simulink model "AdaptiveDilterPrototype"  (R2022b)
settings: Solver=VariableStepAuto  StartTime=0.0  StopTime=10.0  RelTol=1e-3
settings Model: Creator=Ceribro  LastModifiedBy=Ceribro

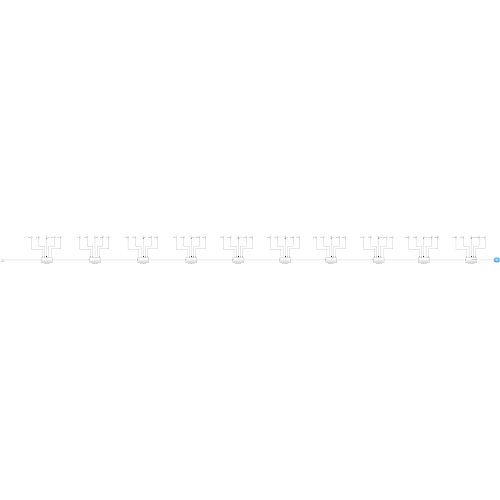
[thumbnail: Simulink's stored preview of the top-level diagram]
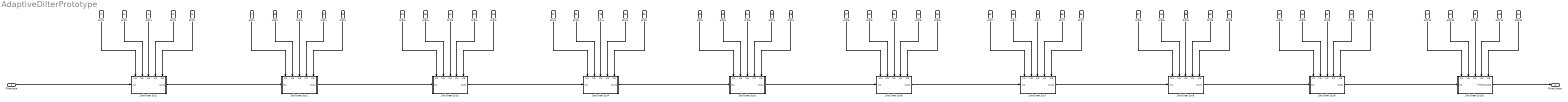
== system AdaptiveDilterPrototype ==
  FilterInput : Inport
  a(2)1 : Inport  Port=2
  b(2)1 : Inport  Port=3
  b(1)1 : Inport  Port=4
  a(3)1 : Inport  Port=5
  b(3)1 : Inport  Port=6
  a(2)2 : Inport  Port=7
  b(2)2 : Inport  Port=8
  b(1)2 : Inport  Port=9
  a(3)2 : Inport  Port=10
  b(3)2 : Inport  Port=11
  a(2)3 : Inport  Port=12
  b(2)3 : Inport  Port=13
  b(1)3 : Inport  Port=14
  a(3)3 : Inport  Port=15
  b(3)3 : Inport  Port=16
  a(2)4 : Inport  Port=17
  b(2)4 : Inport  Port=18
  b(1)4 : Inport  Port=19
  a(3)4 : Inport  Port=20
  b(3)4 : Inport  Port=21
  a(2)5 : Inport  Port=22
  b(2)5 : Inport  Port=23
  b(1)5 : Inport  Port=24
  a(3)5 : Inport  Port=25
  b(3)5 : Inport  Port=26
  a(2)6 : Inport  Port=27
  b(2)6 : Inport  Port=28
  b(1)6 : Inport  Port=29
  a(3)6 : Inport  Port=30
  b(3)6 : Inport  Port=31
  a(2)7 : Inport  Port=32
  b(2)7 : Inport  Port=33
  b(1)7 : Inport  Port=34
  a(3)7 : Inport  Port=35
  b(3)7 : Inport  Port=36
  a(2)8 : Inport  Port=37
  b(2)8 : Inport  Port=38
  b(1)8 : Inport  Port=39
  a(3)8 : Inport  Port=40
  b(3)8 : Inport  Port=41
  a(2)9 : Inport  Port=42
  b(2)9 : Inport  Port=43
  b(1)9 : Inport  Port=44
  a(3)9 : Inport  Port=45
  b(3)9 : Inport  Port=46
  a(2)10 : Inport  Port=47
  b(2)10 : Inport  Port=48
  b(1)10 : Inport  Port=49
  a(3)10 : Inport  Port=50
  b(3)10 : Inport  Port=51
  2nd Order Sys1 : Subsystem
      settings: PortSchema="{\"entries\":[{\"content\":{\"sides\":[{\"content\":{\"connectorIds\":[\"In1\",\"In2\",\"In3\",\"In4\",\"In5\"]},\"type\":\"ConnectorPlacement.EquallySpacedRectSide\",\"uuid\":\"b9dbb1a8-51a6-4b96-96bf-c9da2300ff43\"},{\"content\":{\"connectorIds\":[],\"side\":\"RIGHT\"},\"type\":\"ConnectorPlacement.EquallySpacedRectSide\",\"uuid\":\"4cac1354-1c5d-4db6-b4d6-5d3a283dca26\"},{\"content\":{\"connectorIds\":[\"In6\"],\"side\":\"TOP\"},\"type\":\"ConnectorPlacement.EquallySpacedRectSide\",\"uuid\":\"b7090e22-aad0-44be-a576-af352fa4e03b\"},{\"content\":{\"connectorIds\":[\"Out1\"],\"side\":\"BOTTOM\"},\"type\":\"ConnectorPlacement.EquallySpacedRectSide\",\"uuid\":\"8692f441-cf04-4506-bf52-8e3a9e9e20b6\"}]},\"type\":\"ConnectorPlacement.EquallySpacedConnector\",\"uuid\":\"e0d2a6b7-a198-4ea6-960b-9fb200603ab4\"}],\"packageUris\":[\"http://schema.mathworks.com/mf0/Connector/R2020b\"],\"version\":\"1.0\"}"
  2nd Order Sys10 : Subsystem
      settings: PortSchema="{\"entries\":[{\"content\":{\"sides\":[{\"content\":{\"connectorIds\":[\"In1\",\"In2\",\"In3\",\"In4\",\"In5\"]},\"type\":\"ConnectorPlacement.EquallySpacedRectSide\",\"uuid\":\"b9dbb1a8-51a6-4b96-96bf-c9da2300ff43\"},{\"content\":{\"connectorIds\":[],\"side\":\"RIGHT\"},\"type\":\"ConnectorPlacement.EquallySpacedRectSide\",\"uuid\":\"4cac1354-1c5d-4db6-b4d6-5d3a283dca26\"},{\"content\":{\"connectorIds\":[\"In6\"],\"side\":\"TOP\"},\"type\":\"ConnectorPlacement.EquallySpacedRectSide\",\"uuid\":\"b7090e22-aad0-44be-a576-af352fa4e03b\"},{\"content\":{\"connectorIds\":[\"Out1\"],\"side\":\"BOTTOM\"},\"type\":\"ConnectorPlacement.EquallySpacedRectSide\",\"uuid\":\"8692f441-cf04-4506-bf52-8e3a9e9e20b6\"}]},\"type\":\"ConnectorPlacement.EquallySpacedConnector\",\"uuid\":\"e0d2a6b7-a198-4ea6-960b-9fb200603ab4\"}],\"packageUris\":[\"http://schema.mathworks.com/mf0/Connector/R2020b\"],\"version\":\"1.0\"}"
  2nd Order Sys2 : Subsystem
      settings: PortSchema="{\"entries\":[{\"content\":{\"sides\":[{\"content\":{\"connectorIds\":[\"In1\",\"In2\",\"In3\",\"In4\",\"In5\"]},\"type\":\"ConnectorPlacement.EquallySpacedRectSide\",\"uuid\":\"b9dbb1a8-51a6-4b96-96bf-c9da2300ff43\"},{\"content\":{\"connectorIds\":[],\"side\":\"RIGHT\"},\"type\":\"ConnectorPlacement.EquallySpacedRectSide\",\"uuid\":\"4cac1354-1c5d-4db6-b4d6-5d3a283dca26\"},{\"content\":{\"connectorIds\":[\"In6\"],\"side\":\"TOP\"},\"type\":\"ConnectorPlacement.EquallySpacedRectSide\",\"uuid\":\"b7090e22-aad0-44be-a576-af352fa4e03b\"},{\"content\":{\"connectorIds\":[\"Out1\"],\"side\":\"BOTTOM\"},\"type\":\"ConnectorPlacement.EquallySpacedRectSide\",\"uuid\":\"8692f441-cf04-4506-bf52-8e3a9e9e20b6\"}]},\"type\":\"ConnectorPlacement.EquallySpacedConnector\",\"uuid\":\"e0d2a6b7-a198-4ea6-960b-9fb200603ab4\"}],\"packageUris\":[\"http://schema.mathworks.com/mf0/Connector/R2020b\"],\"version\":\"1.0\"}"
  2nd Order Sys3 : Subsystem
      settings: PortSchema="{\"entries\":[{\"content\":{\"sides\":[{\"content\":{\"connectorIds\":[\"In1\",\"In2\",\"In3\",\"In4\",\"In5\"]},\"type\":\"ConnectorPlacement.EquallySpacedRectSide\",\"uuid\":\"b9dbb1a8-51a6-4b96-96bf-c9da2300ff43\"},{\"content\":{\"connectorIds\":[],\"side\":\"RIGHT\"},\"type\":\"ConnectorPlacement.EquallySpacedRectSide\",\"uuid\":\"4cac1354-1c5d-4db6-b4d6-5d3a283dca26\"},{\"content\":{\"connectorIds\":[\"In6\"],\"side\":\"TOP\"},\"type\":\"ConnectorPlacement.EquallySpacedRectSide\",\"uuid\":\"b7090e22-aad0-44be-a576-af352fa4e03b\"},{\"content\":{\"connectorIds\":[\"Out1\"],\"side\":\"BOTTOM\"},\"type\":\"ConnectorPlacement.EquallySpacedRectSide\",\"uuid\":\"8692f441-cf04-4506-bf52-8e3a9e9e20b6\"}]},\"type\":\"ConnectorPlacement.EquallySpacedConnector\",\"uuid\":\"e0d2a6b7-a198-4ea6-960b-9fb200603ab4\"}],\"packageUris\":[\"http://schema.mathworks.com/mf0/Connector/R2020b\"],\"version\":\"1.0\"}"
  2nd Order Sys4 : Subsystem
      settings: PortSchema="{\"entries\":[{\"content\":{\"sides\":[{\"content\":{\"connectorIds\":[\"In1\",\"In2\",\"In3\",\"In4\",\"In5\"]},\"type\":\"ConnectorPlacement.EquallySpacedRectSide\",\"uuid\":\"b9dbb1a8-51a6-4b96-96bf-c9da2300ff43\"},{\"content\":{\"connectorIds\":[],\"side\":\"RIGHT\"},\"type\":\"ConnectorPlacement.EquallySpacedRectSide\",\"uuid\":\"4cac1354-1c5d-4db6-b4d6-5d3a283dca26\"},{\"content\":{\"connectorIds\":[\"In6\"],\"side\":\"TOP\"},\"type\":\"ConnectorPlacement.EquallySpacedRectSide\",\"uuid\":\"b7090e22-aad0-44be-a576-af352fa4e03b\"},{\"content\":{\"connectorIds\":[\"Out1\"],\"side\":\"BOTTOM\"},\"type\":\"ConnectorPlacement.EquallySpacedRectSide\",\"uuid\":\"8692f441-cf04-4506-bf52-8e3a9e9e20b6\"}]},\"type\":\"ConnectorPlacement.EquallySpacedConnector\",\"uuid\":\"e0d2a6b7-a198-4ea6-960b-9fb200603ab4\"}],\"packageUris\":[\"http://schema.mathworks.com/mf0/Connector/R2020b\"],\"version\":\"1.0\"}"
  2nd Order Sys5 : Subsystem
      settings: PortSchema="{\"entries\":[{\"content\":{\"sides\":[{\"content\":{\"connectorIds\":[\"In1\",\"In2\",\"In3\",\"In4\",\"In5\"]},\"type\":\"ConnectorPlacement.EquallySpacedRectSide\",\"uuid\":\"b9dbb1a8-51a6-4b96-96bf-c9da2300ff43\"},{\"content\":{\"connectorIds\":[],\"side\":\"RIGHT\"},\"type\":\"ConnectorPlacement.EquallySpacedRectSide\",\"uuid\":\"4cac1354-1c5d-4db6-b4d6-5d3a283dca26\"},{\"content\":{\"connectorIds\":[\"In6\"],\"side\":\"TOP\"},\"type\":\"ConnectorPlacement.EquallySpacedRectSide\",\"uuid\":\"b7090e22-aad0-44be-a576-af352fa4e03b\"},{\"content\":{\"connectorIds\":[\"Out1\"],\"side\":\"BOTTOM\"},\"type\":\"ConnectorPlacement.EquallySpacedRectSide\",\"uuid\":\"8692f441-cf04-4506-bf52-8e3a9e9e20b6\"}]},\"type\":\"ConnectorPlacement.EquallySpacedConnector\",\"uuid\":\"e0d2a6b7-a198-4ea6-960b-9fb200603ab4\"}],\"packageUris\":[\"http://schema.mathworks.com/mf0/Connector/R2020b\"],\"version\":\"1.0\"}"
  2nd Order Sys6 : Subsystem
      settings: PortSchema="{\"entries\":[{\"content\":{\"sides\":[{\"content\":{\"connectorIds\":[\"In1\",\"In2\",\"In3\",\"In4\",\"In5\"]},\"type\":\"ConnectorPlacement.EquallySpacedRectSide\",\"uuid\":\"b9dbb1a8-51a6-4b96-96bf-c9da2300ff43\"},{\"content\":{\"connectorIds\":[],\"side\":\"RIGHT\"},\"type\":\"ConnectorPlacement.EquallySpacedRectSide\",\"uuid\":\"4cac1354-1c5d-4db6-b4d6-5d3a283dca26\"},{\"content\":{\"connectorIds\":[\"In6\"],\"side\":\"TOP\"},\"type\":\"ConnectorPlacement.EquallySpacedRectSide\",\"uuid\":\"b7090e22-aad0-44be-a576-af352fa4e03b\"},{\"content\":{\"connectorIds\":[\"Out1\"],\"side\":\"BOTTOM\"},\"type\":\"ConnectorPlacement.EquallySpacedRectSide\",\"uuid\":\"8692f441-cf04-4506-bf52-8e3a9e9e20b6\"}]},\"type\":\"ConnectorPlacement.EquallySpacedConnector\",\"uuid\":\"e0d2a6b7-a198-4ea6-960b-9fb200603ab4\"}],\"packageUris\":[\"http://schema.mathworks.com/mf0/Connector/R2020b\"],\"version\":\"1.0\"}"
  2nd Order Sys7 : Subsystem
      settings: PortSchema="{\"entries\":[{\"content\":{\"sides\":[{\"content\":{\"connectorIds\":[\"In1\",\"In2\",\"In3\",\"In4\",\"In5\"]},\"type\":\"ConnectorPlacement.EquallySpacedRectSide\",\"uuid\":\"b9dbb1a8-51a6-4b96-96bf-c9da2300ff43\"},{\"content\":{\"connectorIds\":[],\"side\":\"RIGHT\"},\"type\":\"ConnectorPlacement.EquallySpacedRectSide\",\"uuid\":\"4cac1354-1c5d-4db6-b4d6-5d3a283dca26\"},{\"content\":{\"connectorIds\":[\"In6\"],\"side\":\"TOP\"},\"type\":\"ConnectorPlacement.EquallySpacedRectSide\",\"uuid\":\"b7090e22-aad0-44be-a576-af352fa4e03b\"},{\"content\":{\"connectorIds\":[\"Out1\"],\"side\":\"BOTTOM\"},\"type\":\"ConnectorPlacement.EquallySpacedRectSide\",\"uuid\":\"8692f441-cf04-4506-bf52-8e3a9e9e20b6\"}]},\"type\":\"ConnectorPlacement.EquallySpacedConnector\",\"uuid\":\"e0d2a6b7-a198-4ea6-960b-9fb200603ab4\"}],\"packageUris\":[\"http://schema.mathworks.com/mf0/Connector/R2020b\"],\"version\":\"1.0\"}"
  2nd Order Sys8 : Subsystem
      settings: PortSchema="{\"entries\":[{\"content\":{\"sides\":[{\"content\":{\"connectorIds\":[\"In1\",\"In2\",\"In3\",\"In4\",\"In5\"]},\"type\":\"ConnectorPlacement.EquallySpacedRectSide\",\"uuid\":\"b9dbb1a8-51a6-4b96-96bf-c9da2300ff43\"},{\"content\":{\"connectorIds\":[],\"side\":\"RIGHT\"},\"type\":\"ConnectorPlacement.EquallySpacedRectSide\",\"uuid\":\"4cac1354-1c5d-4db6-b4d6-5d3a283dca26\"},{\"content\":{\"connectorIds\":[\"In6\"],\"side\":\"TOP\"},\"type\":\"ConnectorPlacement.EquallySpacedRectSide\",\"uuid\":\"b7090e22-aad0-44be-a576-af352fa4e03b\"},{\"content\":{\"connectorIds\":[\"Out1\"],\"side\":\"BOTTOM\"},\"type\":\"ConnectorPlacement.EquallySpacedRectSide\",\"uuid\":\"8692f441-cf04-4506-bf52-8e3a9e9e20b6\"}]},\"type\":\"ConnectorPlacement.EquallySpacedConnector\",\"uuid\":\"e0d2a6b7-a198-4ea6-960b-9fb200603ab4\"}],\"packageUris\":[\"http://schema.mathworks.com/mf0/Connector/R2020b\"],\"version\":\"1.0\"}"
  2nd Order Sys9 : Subsystem
      settings: PortSchema="{\"entries\":[{\"content\":{\"sides\":[{\"content\":{\"connectorIds\":[\"In1\",\"In2\",\"In3\",\"In4\",\"In5\"]},\"type\":\"ConnectorPlacement.EquallySpacedRectSide\",\"uuid\":\"b9dbb1a8-51a6-4b96-96bf-c9da2300ff43\"},{\"content\":{\"connectorIds\":[],\"side\":\"RIGHT\"},\"type\":\"ConnectorPlacement.EquallySpacedRectSide\",\"uuid\":\"4cac1354-1c5d-4db6-b4d6-5d3a283dca26\"},{\"content\":{\"connectorIds\":[\"In6\"],\"side\":\"TOP\"},\"type\":\"ConnectorPlacement.EquallySpacedRectSide\",\"uuid\":\"b7090e22-aad0-44be-a576-af352fa4e03b\"},{\"content\":{\"connectorIds\":[\"Out1\"],\"side\":\"BOTTOM\"},\"type\":\"ConnectorPlacement.EquallySpacedRectSide\",\"uuid\":\"8692f441-cf04-4506-bf52-8e3a9e9e20b6\"}]},\"type\":\"ConnectorPlacement.EquallySpacedConnector\",\"uuid\":\"e0d2a6b7-a198-4ea6-960b-9fb200603ab4\"}],\"packageUris\":[\"http://schema.mathworks.com/mf0/Connector/R2020b\"],\"version\":\"1.0\"}"
  FilterOutput : Outport
  wires:
  a(2)1/1 -> 2nd Order Sys1/1(In1)
  b(2)1/1 -> 2nd Order Sys1/4(In2)
  b(1)1/1 -> 2nd Order Sys1/3(In3)
  FilterInput/1 -> 2nd Order Sys1/6(In4)
  a(3)1/1 -> 2nd Order Sys1/2(In5)
  b(3)1/1 -> 2nd Order Sys1/5(In6)
  a(3)2/1 -> 2nd Order Sys2/2(In5)
  2nd Order Sys1/1(Out1) -> 2nd Order Sys2/6(In4)
  b(2)2/1 -> 2nd Order Sys2/4(In2)
  b(1)2/1 -> 2nd Order Sys2/3(In3)
  a(2)2/1 -> 2nd Order Sys2/1(In1)
  b(3)2/1 -> 2nd Order Sys2/5(In6)
  a(2)3/1 -> 2nd Order Sys3/1(In1)
  b(2)3/1 -> 2nd Order Sys3/4(In2)
  b(3)3/1 -> 2nd Order Sys3/5(In6)
  a(3)3/1 -> 2nd Order Sys3/2(In5)
  2nd Order Sys2/1(Out1) -> 2nd Order Sys3/6(In4)
  b(1)3/1 -> 2nd Order Sys3/3(In3)
  b(2)4/1 -> 2nd Order Sys4/4(In2)
  b(3)4/1 -> 2nd Order Sys4/5(In6)
  a(2)4/1 -> 2nd Order Sys4/1(In1)
  a(3)4/1 -> 2nd Order Sys4/2(In5)
  2nd Order Sys3/1(Out1) -> 2nd Order Sys4/6(In4)
  b(1)4/1 -> 2nd Order Sys4/3(In3)
  b(2)5/1 -> 2nd Order Sys5/4(In2)
  b(3)5/1 -> 2nd Order Sys5/5(In6)
  a(2)5/1 -> 2nd Order Sys5/1(In1)
  a(3)5/1 -> 2nd Order Sys5/2(In5)
  2nd Order Sys4/1(Out1) -> 2nd Order Sys5/6(In4)
  b(1)5/1 -> 2nd Order Sys5/3(In3)
  2nd Order Sys5/1(Out1) -> 2nd Order Sys6/6(In4)
  a(2)6/1 -> 2nd Order Sys6/1(In1)
  b(1)6/1 -> 2nd Order Sys6/3(In3)
  b(3)6/1 -> 2nd Order Sys6/5(In6)
  b(2)6/1 -> 2nd Order Sys6/4(In2)
  a(3)6/1 -> 2nd Order Sys6/2(In5)
  2nd Order Sys6/1(Out1) -> 2nd Order Sys7/6(In4)
  a(2)7/1 -> 2nd Order Sys7/1(In1)
  b(1)7/1 -> 2nd Order Sys7/3(In3)
  b(3)7/1 -> 2nd Order Sys7/5(In6)
  b(2)7/1 -> 2nd Order Sys7/4(In2)
  a(3)7/1 -> 2nd Order Sys7/2(In5)
  2nd Order Sys7/1(Out1) -> 2nd Order Sys8/6(In4)
  a(2)8/1 -> 2nd Order Sys8/1(In1)
  b(1)8/1 -> 2nd Order Sys8/3(In3)
  b(3)8/1 -> 2nd Order Sys8/5(In6)
  b(2)8/1 -> 2nd Order Sys8/4(In2)
  a(3)8/1 -> 2nd Order Sys8/2(In5)
  2nd Order Sys8/1(Out1) -> 2nd Order Sys9/6(In4)
  a(2)9/1 -> 2nd Order Sys9/1(In1)
  b(1)9/1 -> 2nd Order Sys9/3(In3)
  b(3)9/1 -> 2nd Order Sys9/5(In6)
  b(2)9/1 -> 2nd Order Sys9/4(In2)
  a(3)9/1 -> 2nd Order Sys9/2(In5)
  2nd Order Sys9/1(Out1) -> 2nd Order Sys10/6(In4)
  a(2)10/1 -> 2nd Order Sys10/1(In1)
  b(1)10/1 -> 2nd Order Sys10/3(In3)
  b(3)10/1 -> 2nd Order Sys10/5(In6)
  b(2)10/1 -> 2nd Order Sys10/4(In2)
  a(3)10/1 -> 2nd Order Sys10/2(In5)
  2nd Order Sys10/1(FilterOutput) -> FilterOutput/1

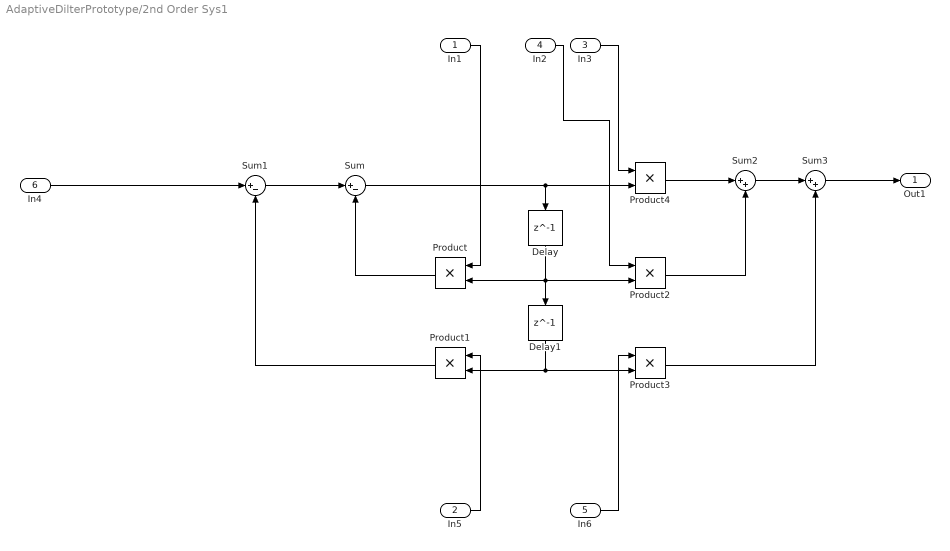
== system AdaptiveDilterPrototype/2nd Order Sys1 ==
  In1 : Inport
  In5 : Inport  Port=2
  In3 : Inport  Port=3
  In2 : Inport  Port=4
  In6 : Inport  Port=5
  In4 : Inport  Port=6
  Delay : Delay  DelayLength=1  InitialCondition=0
  Delay1 : Delay  DelayLength=1  InitialCondition=0
  Product{,1..4} (5 alike) : Product
  Sum : Sum  Inputs=|+-
  Sum1 : Sum  Inputs=|+-
  Sum2 : Sum  Inputs=|++
  Sum3 : Sum  Inputs=|++
  Out1 : Outport
  wires:
  Sum1/1 -> Sum/1
  Product4/1 -> Sum2/1
  Delay1/1 -> Product3/2, Product1/2
  Product1/1 -> Sum1/2
  Product/1 -> Sum/2
  Product2/1 -> Sum2/2
  Sum2/1 -> Sum3/1
  Sum/1 -> Product4/2, Delay/1
  Delay/1 -> Product2/2, Product/2, Delay1/1
  Product3/1 -> Sum3/2
  In5/1 -> Product1/1
  In4/1 -> Sum1/1
  In6/1 -> Product3/1
  In3/1 -> Product4/1
  In2/1 -> Product2/1
  Sum3/1 -> Out1/1
  In1/1 -> Product/1

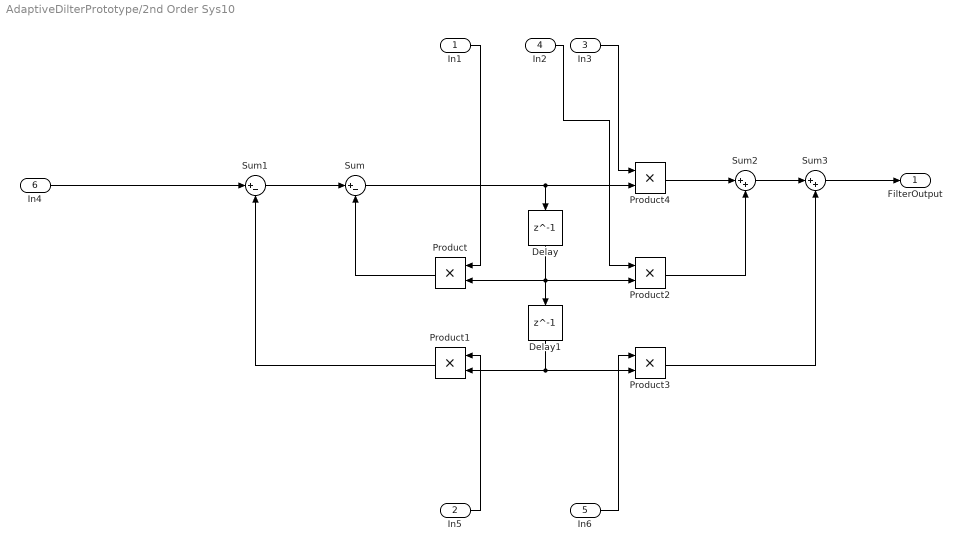
== system AdaptiveDilterPrototype/2nd Order Sys10 ==
  In1 : Inport
  In5 : Inport  Port=2
  In3 : Inport  Port=3
  In2 : Inport  Port=4
  In6 : Inport  Port=5
  In4 : Inport  Port=6
  Delay : Delay  DelayLength=1  InitialCondition=0
  Delay1 : Delay  DelayLength=1  InitialCondition=0
  Product{,1..4} (5 alike) : Product
  Sum : Sum  Inputs=|+-
  Sum1 : Sum  Inputs=|+-
  Sum2 : Sum  Inputs=|++
  Sum3 : Sum  Inputs=|++
  FilterOutput : Outport
  wires:
  Sum1/1 -> Sum/1
  Product4/1 -> Sum2/1
  Delay1/1 -> Product3/2, Product1/2
  Product1/1 -> Sum1/2
  Product/1 -> Sum/2
  Product2/1 -> Sum2/2
  Sum2/1 -> Sum3/1
  Sum/1 -> Product4/2, Delay/1
  Delay/1 -> Product2/2, Product/2, Delay1/1
  Product3/1 -> Sum3/2
  In5/1 -> Product1/1
  In4/1 -> Sum1/1
  In6/1 -> Product3/1
  In3/1 -> Product4/1
  In2/1 -> Product2/1
  Sum3/1 -> FilterOutput/1
  In1/1 -> Product/1

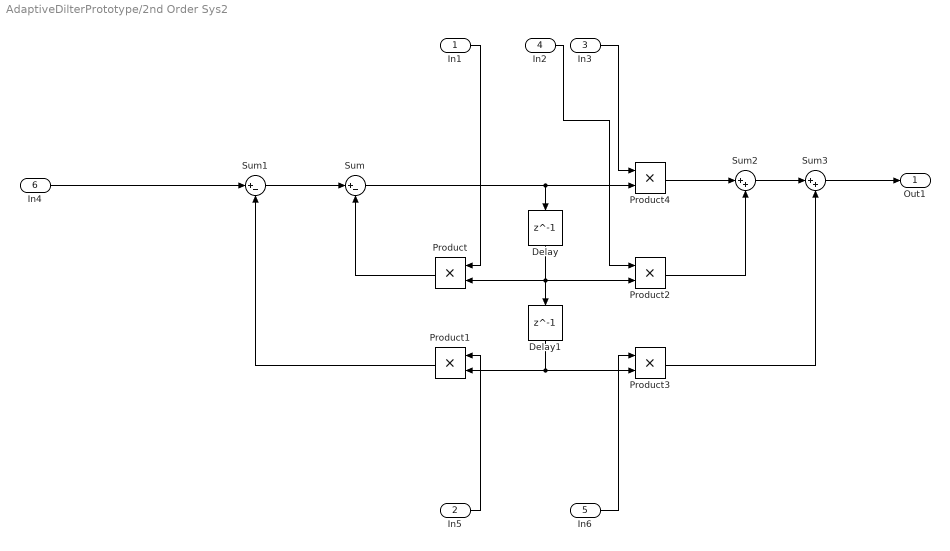
== system AdaptiveDilterPrototype/2nd Order Sys2 ==
  In1 : Inport
  In5 : Inport  Port=2
  In3 : Inport  Port=3
  In2 : Inport  Port=4
  In6 : Inport  Port=5
  In4 : Inport  Port=6
  Delay : Delay  DelayLength=1  InitialCondition=0
  Delay1 : Delay  DelayLength=1  InitialCondition=0
  Product{,1..4} (5 alike) : Product
  Sum : Sum  Inputs=|+-
  Sum1 : Sum  Inputs=|+-
  Sum2 : Sum  Inputs=|++
  Sum3 : Sum  Inputs=|++
  Out1 : Outport
  wires:
  Sum1/1 -> Sum/1
  Product4/1 -> Sum2/1
  Delay1/1 -> Product3/2, Product1/2
  Product1/1 -> Sum1/2
  Product/1 -> Sum/2
  Product2/1 -> Sum2/2
  Sum2/1 -> Sum3/1
  Sum/1 -> Product4/2, Delay/1
  Delay/1 -> Product2/2, Product/2, Delay1/1
  Product3/1 -> Sum3/2
  In5/1 -> Product1/1
  In4/1 -> Sum1/1
  In6/1 -> Product3/1
  In3/1 -> Product4/1
  In2/1 -> Product2/1
  Sum3/1 -> Out1/1
  In1/1 -> Product/1

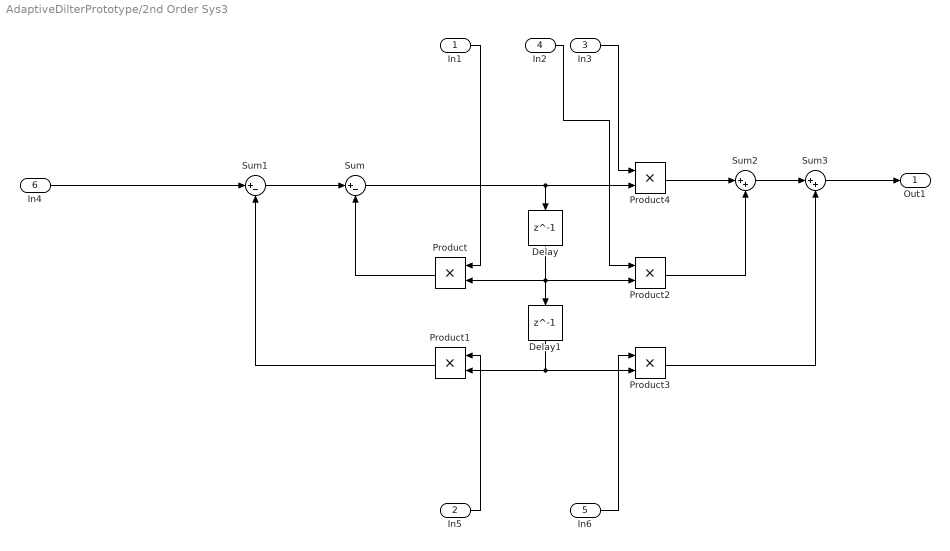
== system AdaptiveDilterPrototype/2nd Order Sys3 ==
  In1 : Inport
  In5 : Inport  Port=2
  In3 : Inport  Port=3
  In2 : Inport  Port=4
  In6 : Inport  Port=5
  In4 : Inport  Port=6
  Delay : Delay  DelayLength=1  InitialCondition=0
  Delay1 : Delay  DelayLength=1  InitialCondition=0
  Product{,1..4} (5 alike) : Product
  Sum : Sum  Inputs=|+-
  Sum1 : Sum  Inputs=|+-
  Sum2 : Sum  Inputs=|++
  Sum3 : Sum  Inputs=|++
  Out1 : Outport
  wires:
  Sum1/1 -> Sum/1
  Product4/1 -> Sum2/1
  Delay1/1 -> Product3/2, Product1/2
  Product1/1 -> Sum1/2
  Product/1 -> Sum/2
  Product2/1 -> Sum2/2
  Sum2/1 -> Sum3/1
  Sum/1 -> Product4/2, Delay/1
  Delay/1 -> Product2/2, Product/2, Delay1/1
  Product3/1 -> Sum3/2
  In5/1 -> Product1/1
  In4/1 -> Sum1/1
  In6/1 -> Product3/1
  In3/1 -> Product4/1
  In2/1 -> Product2/1
  Sum3/1 -> Out1/1
  In1/1 -> Product/1

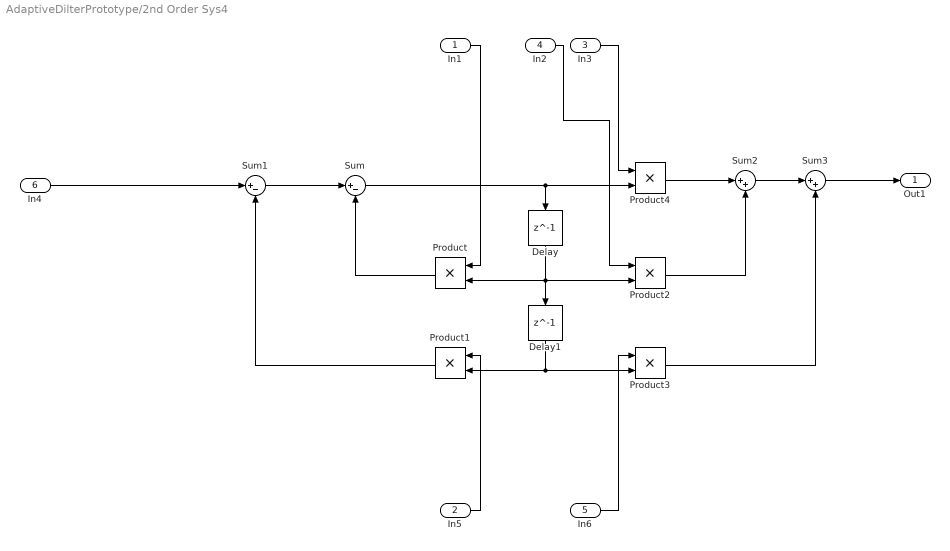
== system AdaptiveDilterPrototype/2nd Order Sys4 ==
  In1 : Inport
  In5 : Inport  Port=2
  In3 : Inport  Port=3
  In2 : Inport  Port=4
  In6 : Inport  Port=5
  In4 : Inport  Port=6
  Delay : Delay  DelayLength=1  InitialCondition=0
  Delay1 : Delay  DelayLength=1  InitialCondition=0
  Product{,1..4} (5 alike) : Product
  Sum : Sum  Inputs=|+-
  Sum1 : Sum  Inputs=|+-
  Sum2 : Sum  Inputs=|++
  Sum3 : Sum  Inputs=|++
  Out1 : Outport
  wires:
  Sum1/1 -> Sum/1
  Product4/1 -> Sum2/1
  Delay1/1 -> Product3/2, Product1/2
  Product1/1 -> Sum1/2
  Product/1 -> Sum/2
  Product2/1 -> Sum2/2
  Sum2/1 -> Sum3/1
  Sum/1 -> Product4/2, Delay/1
  Delay/1 -> Product2/2, Product/2, Delay1/1
  Product3/1 -> Sum3/2
  In5/1 -> Product1/1
  In4/1 -> Sum1/1
  In6/1 -> Product3/1
  In3/1 -> Product4/1
  In2/1 -> Product2/1
  Sum3/1 -> Out1/1
  In1/1 -> Product/1

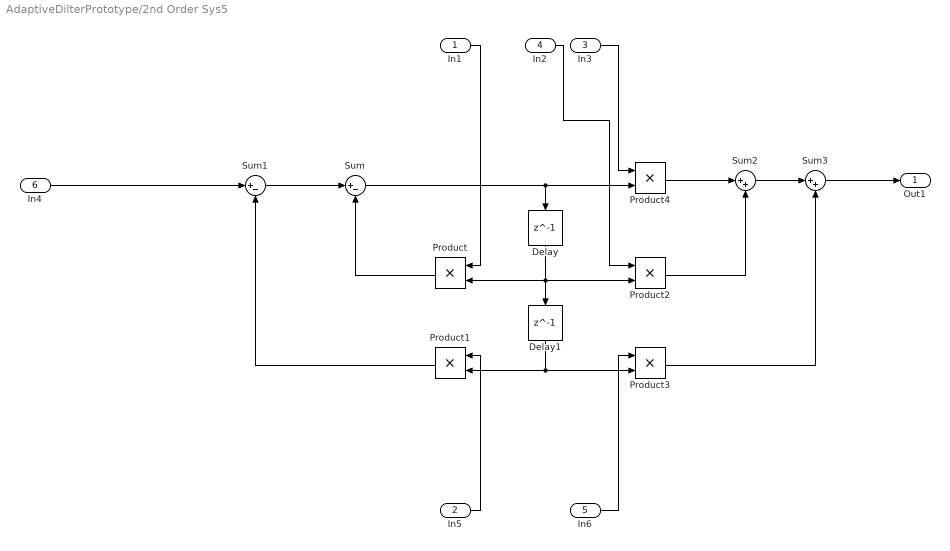
== system AdaptiveDilterPrototype/2nd Order Sys5 ==
  In1 : Inport
  In5 : Inport  Port=2
  In3 : Inport  Port=3
  In2 : Inport  Port=4
  In6 : Inport  Port=5
  In4 : Inport  Port=6
  Delay : Delay  DelayLength=1  InitialCondition=0
  Delay1 : Delay  DelayLength=1  InitialCondition=0
  Product{,1..4} (5 alike) : Product
  Sum : Sum  Inputs=|+-
  Sum1 : Sum  Inputs=|+-
  Sum2 : Sum  Inputs=|++
  Sum3 : Sum  Inputs=|++
  Out1 : Outport
  wires:
  Sum1/1 -> Sum/1
  Product4/1 -> Sum2/1
  Delay1/1 -> Product3/2, Product1/2
  Product1/1 -> Sum1/2
  Product/1 -> Sum/2
  Product2/1 -> Sum2/2
  Sum2/1 -> Sum3/1
  Sum/1 -> Product4/2, Delay/1
  Delay/1 -> Product2/2, Product/2, Delay1/1
  Product3/1 -> Sum3/2
  In5/1 -> Product1/1
  In4/1 -> Sum1/1
  In6/1 -> Product3/1
  In3/1 -> Product4/1
  In2/1 -> Product2/1
  Sum3/1 -> Out1/1
  In1/1 -> Product/1

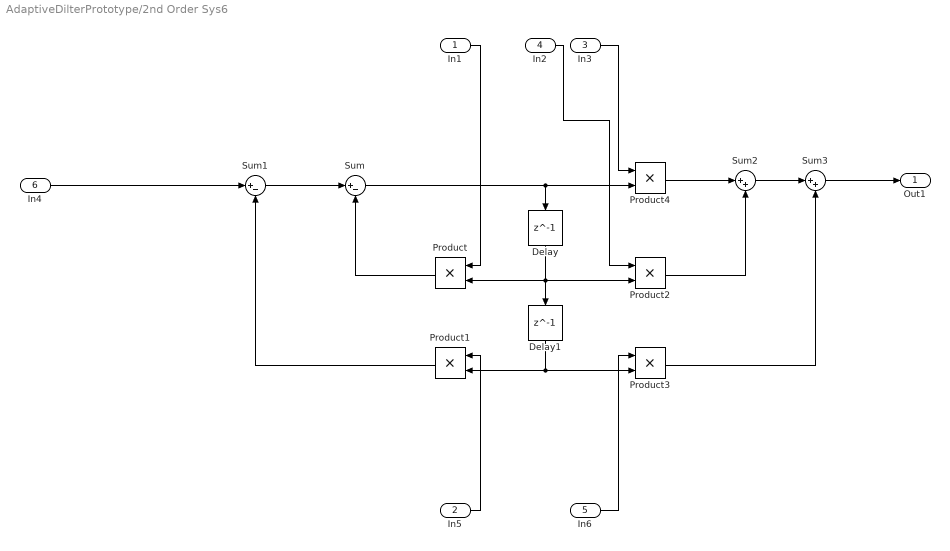
== system AdaptiveDilterPrototype/2nd Order Sys6 ==
  In1 : Inport
  In5 : Inport  Port=2
  In3 : Inport  Port=3
  In2 : Inport  Port=4
  In6 : Inport  Port=5
  In4 : Inport  Port=6
  Delay : Delay  DelayLength=1  InitialCondition=0
  Delay1 : Delay  DelayLength=1  InitialCondition=0
  Product{,1..4} (5 alike) : Product
  Sum : Sum  Inputs=|+-
  Sum1 : Sum  Inputs=|+-
  Sum2 : Sum  Inputs=|++
  Sum3 : Sum  Inputs=|++
  Out1 : Outport
  wires:
  Sum1/1 -> Sum/1
  Product4/1 -> Sum2/1
  Delay1/1 -> Product3/2, Product1/2
  Product1/1 -> Sum1/2
  Product/1 -> Sum/2
  Product2/1 -> Sum2/2
  Sum2/1 -> Sum3/1
  Sum/1 -> Product4/2, Delay/1
  Delay/1 -> Product2/2, Product/2, Delay1/1
  Product3/1 -> Sum3/2
  In5/1 -> Product1/1
  In4/1 -> Sum1/1
  In6/1 -> Product3/1
  In3/1 -> Product4/1
  In2/1 -> Product2/1
  Sum3/1 -> Out1/1
  In1/1 -> Product/1

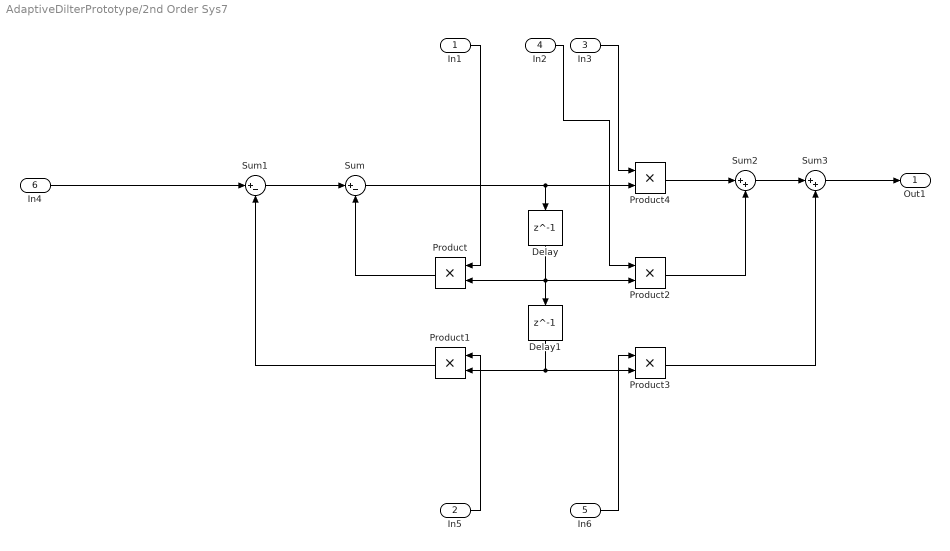
== system AdaptiveDilterPrototype/2nd Order Sys7 ==
  In1 : Inport
  In5 : Inport  Port=2
  In3 : Inport  Port=3
  In2 : Inport  Port=4
  In6 : Inport  Port=5
  In4 : Inport  Port=6
  Delay : Delay  DelayLength=1  InitialCondition=0
  Delay1 : Delay  DelayLength=1  InitialCondition=0
  Product{,1..4} (5 alike) : Product
  Sum : Sum  Inputs=|+-
  Sum1 : Sum  Inputs=|+-
  Sum2 : Sum  Inputs=|++
  Sum3 : Sum  Inputs=|++
  Out1 : Outport
  wires:
  Sum1/1 -> Sum/1
  Product4/1 -> Sum2/1
  Delay1/1 -> Product3/2, Product1/2
  Product1/1 -> Sum1/2
  Product/1 -> Sum/2
  Product2/1 -> Sum2/2
  Sum2/1 -> Sum3/1
  Sum/1 -> Product4/2, Delay/1
  Delay/1 -> Product2/2, Product/2, Delay1/1
  Product3/1 -> Sum3/2
  In5/1 -> Product1/1
  In4/1 -> Sum1/1
  In6/1 -> Product3/1
  In3/1 -> Product4/1
  In2/1 -> Product2/1
  Sum3/1 -> Out1/1
  In1/1 -> Product/1

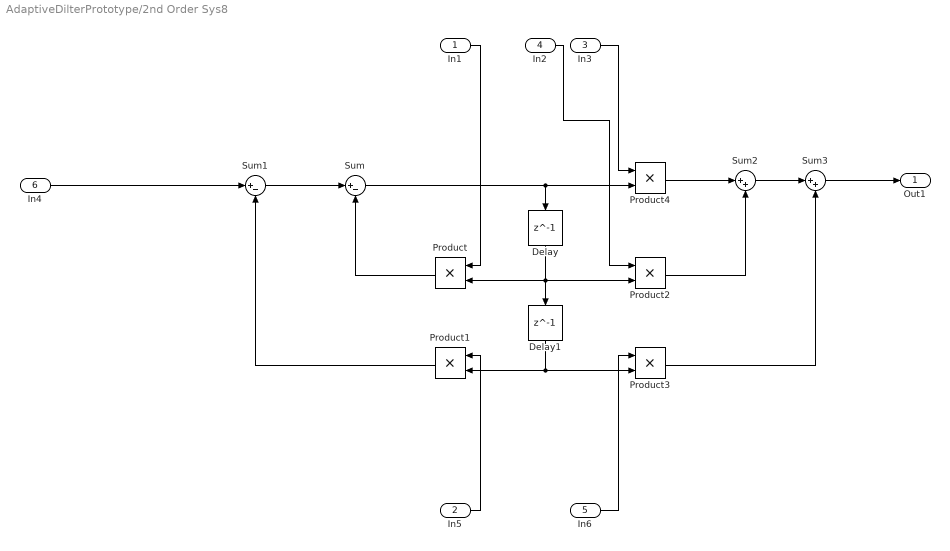
== system AdaptiveDilterPrototype/2nd Order Sys8 ==
  In1 : Inport
  In5 : Inport  Port=2
  In3 : Inport  Port=3
  In2 : Inport  Port=4
  In6 : Inport  Port=5
  In4 : Inport  Port=6
  Delay : Delay  DelayLength=1  InitialCondition=0
  Delay1 : Delay  DelayLength=1  InitialCondition=0
  Product{,1..4} (5 alike) : Product
  Sum : Sum  Inputs=|+-
  Sum1 : Sum  Inputs=|+-
  Sum2 : Sum  Inputs=|++
  Sum3 : Sum  Inputs=|++
  Out1 : Outport
  wires:
  Sum1/1 -> Sum/1
  Product4/1 -> Sum2/1
  Delay1/1 -> Product3/2, Product1/2
  Product1/1 -> Sum1/2
  Product/1 -> Sum/2
  Product2/1 -> Sum2/2
  Sum2/1 -> Sum3/1
  Sum/1 -> Product4/2, Delay/1
  Delay/1 -> Product2/2, Product/2, Delay1/1
  Product3/1 -> Sum3/2
  In5/1 -> Product1/1
  In4/1 -> Sum1/1
  In6/1 -> Product3/1
  In3/1 -> Product4/1
  In2/1 -> Product2/1
  Sum3/1 -> Out1/1
  In1/1 -> Product/1

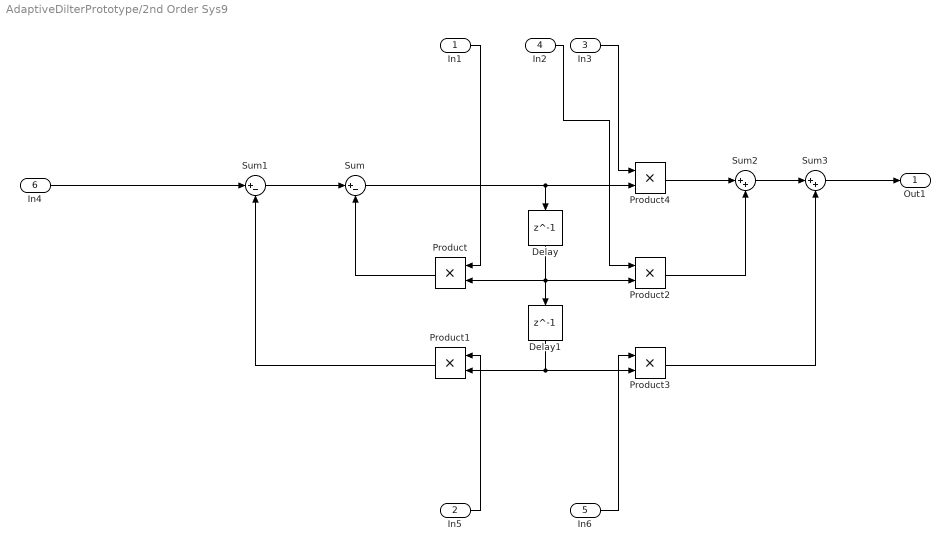
== system AdaptiveDilterPrototype/2nd Order Sys9 ==
  In1 : Inport
  In5 : Inport  Port=2
  In3 : Inport  Port=3
  In2 : Inport  Port=4
  In6 : Inport  Port=5
  In4 : Inport  Port=6
  Delay : Delay  DelayLength=1  InitialCondition=0
  Delay1 : Delay  DelayLength=1  InitialCondition=0
  Product{,1..4} (5 alike) : Product
  Sum : Sum  Inputs=|+-
  Sum1 : Sum  Inputs=|+-
  Sum2 : Sum  Inputs=|++
  Sum3 : Sum  Inputs=|++
  Out1 : Outport
  wires:
  Sum1/1 -> Sum/1
  Product4/1 -> Sum2/1
  Delay1/1 -> Product3/2, Product1/2
  Product1/1 -> Sum1/2
  Product/1 -> Sum/2
  Product2/1 -> Sum2/2
  Sum2/1 -> Sum3/1
  Sum/1 -> Product4/2, Delay/1
  Delay/1 -> Product2/2, Product/2, Delay1/1
  Product3/1 -> Sum3/2
  In5/1 -> Product1/1
  In4/1 -> Sum1/1
  In6/1 -> Product3/1
  In3/1 -> Product4/1
  In2/1 -> Product2/1
  Sum3/1 -> Out1/1
  In1/1 -> Product/1
